simulink model "Model_example"  (R2015a)
settings: Solver=ode45  StartTime=0.0  StopTime=10.0  RelTol=1e-3
settings Model: Creator=shizue  LastModifiedBy=shizue
settings DataIOCC: ExternalInput=[t, u1, u2]

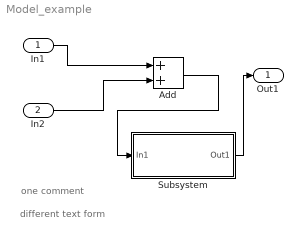
== system Model_example ==
  note: different text form
  note: one comment
  In1 : Inport
  In2 : Inport  Port=2
  Add : Sum
  Subsystem : Subsystem
  Out1 : Outport
  wires:
  In2/1 -> Add/2
  In1/1 -> Add/1
  Add/1 -> Subsystem/1(In1)
  Subsystem/1(Out1) -> Out1/1

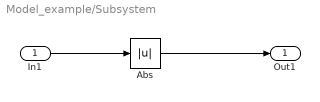
== system Model_example/Subsystem ==
  In1 : Inport
  Abs : Abs
  Out1 : Outport
  wires:
  In1/1 -> Abs/1
  Abs/1 -> Out1/1
